simulink model "saturation"  (R2024b)
settings: Solver=VariableStepAuto  StartTime=0.0  StopTime=10.0  RelTol=1e-3
settings Model: Creator=woutlyen  LastModifiedBy=woutlyen

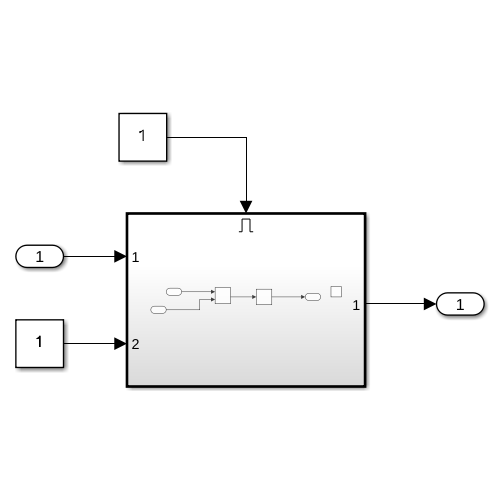
[thumbnail: Simulink's stored preview of the top-level diagram]
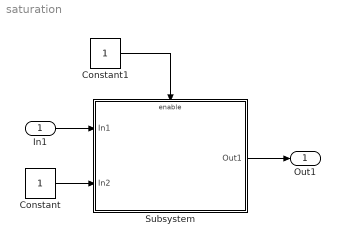
== system saturation ==
  In1 : Inport  OutDataTypeStr=fixdt(1,24,23)
  Constant : Constant  OutDataTypeStr=fixdt(1,27,23)
  Constant1 : Constant  OutDataTypeStr=boolean
  Subsystem : Subsystem
  Out1 : Outport
  wires:
  In1/1 -> Subsystem/1(In1)
  Constant/1 -> Subsystem/2(In2)
  Subsystem/1(Out1) -> Out1/1
  Constant1/1 -> Subsystem/Enable

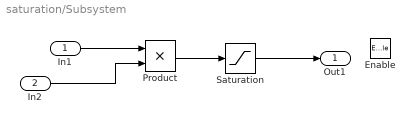
== system saturation/Subsystem ==
  In1 : Inport
  In2 : Inport  Port=2
  Enable : EnablePort
  Product : Product
  Saturation : Saturate  UpperLimit=1  LowerLimit=-1  OutDataTypeStr=fixdt(1,24,23)
  Out1 : Outport
  wires:
  Saturation/1 -> Out1/1
  In2/1 -> Product/2
  Product/1 -> Saturation/1
  In1/1 -> Product/1
